simulink model "wrapper_template_model"  (R2022b)
settings: Solver=FixedStepDiscrete  StartTime=0.0  StopTime=10.0  FixedStep=1/ SCHED_LOOP_RATE  RelTol=1e-3
settings Model: ParamWorkspaceSource=ReferencedWorkspace  Creator=joseph  LastModifiedBy=joseph
settings OptimizationCC: EnhancedBackFolding=on  PassReuseOutputArgsAs=Individual arguments  ZeroExternalMemoryAtStartup=off  ZeroInternalMemoryAtStartup=off  OptimizeBlockOrder=speed  DifferentSizesBufferReuse=on  OptimizationCustomize=off  EfficientTunableParamExpr=on
settings DebuggingCC: ParameterTunabilityLossMsg=error
settings HardwareCC: ProdBitPerPointer=32  ProdBitPerSizeT=32  ProdBitPerPtrDiffT=32  ProdLargestAtomicInteger=Long  ProdLargestAtomicFloat=Double  ProdWordSize=32  ProdHWDeviceType=ARM Compatible->ARM Cortex-M
settings SFSimCC: MATLABDynamicMemAlloc=off
settings RTWCC: Description=Embedded Coder  SystemTargetFile=ert.tlc  GenCodeOnly=on  PackageGeneratedCodeAndArtifacts=on  TemplateMakefile=ert_default_tmf  TargetLang=C++
settings CodeAppCC: ForceParamTrailComments=on  IgnoreCustomStorageClasses=off  OperatorAnnotations=on  SimulinkDataObjDesc=on  SFDataObjDesc=on  InsertBlockDesc=on
settings ERTTargetCC: TargetLangStandard=C++11 (ISO)  GenerateSampleERTMain=on  CodeInterfacePackaging=C++ class  RootIOFormat=Structure reference  ERTCustomFileTemplate=example_file_process.tlc

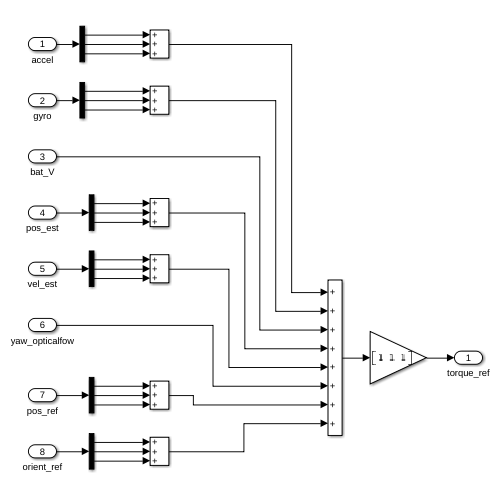
[thumbnail: Simulink's stored preview of the top-level diagram]
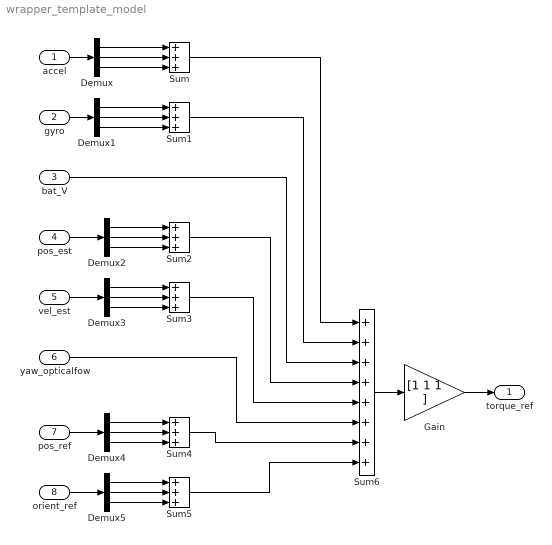
== system wrapper_template_model ==
  accel : Inport  OutDataTypeStr=single
  gyro : Inport  Port=2  OutDataTypeStr=single
  bat_V : Inport  Port=3  OutDataTypeStr=single
  pos_est : Inport  Port=4  OutDataTypeStr=single
  vel_est : Inport  Port=5  OutDataTypeStr=single
  yaw_opticalfow : Inport  Port=6  OutDataTypeStr=single
  pos_ref : Inport  Port=7  OutDataTypeStr=single
  orient_ref : Inport  Port=8  OutDataTypeStr=single
  Demux{,1..5} (6 alike) : Demux  Outputs=3
  Gain : Gain  Gain=[1 1 1 ]
  Sum{,1..5} (6 alike) : Sum  Inputs=+++
  Sum6 : Sum  Inputs=++++++++
  torque_ref : Outport  OutDataTypeStr=single
  wires:
  accel/1 -> Demux/1
  gyro/1 -> Demux1/1
  bat_V/1 -> Sum6/3
  Demux/1 -> Sum/1
  Demux/2 -> Sum/2
  Demux/3 -> Sum/3
  Demux1/1 -> Sum1/1
  Demux1/2 -> Sum1/2
  Demux1/3 -> Sum1/3
  Demux2/3 -> Sum2/3
  Demux2/2 -> Sum2/2
  Demux2/1 -> Sum2/1
  pos_est/1 -> Demux2/1
  vel_est/1 -> Demux3/1
  Demux3/1 -> Sum3/1
  Demux3/2 -> Sum3/2
  Demux3/3 -> Sum3/3
  yaw_opticalfow/1 -> Sum6/6
  Demux5/3 -> Sum5/3
  Demux5/2 -> Sum5/2
  Demux5/1 -> Sum5/1
  orient_ref/1 -> Demux5/1
  pos_ref/1 -> Demux4/1
  Demux4/1 -> Sum4/1
  Demux4/2 -> Sum4/2
  Demux4/3 -> Sum4/3
  Sum6/1 -> Gain/1
  Sum5/1 -> Sum6/8
  Sum4/1 -> Sum6/7
  Sum3/1 -> Sum6/5
  Sum2/1 -> Sum6/4
  Sum1/1 -> Sum6/2
  Sum/1 -> Sum6/1
  Gain/1 -> torque_ref/1
